simulink model "Mdl_wFuelLidOpen"  (R2024b)
settings: Solver=FixedStepDiscrete  StartTime=0.0  StopTime=10.0  FixedStep=0.1  RelTol=1e-3  EnableMultiTasking=on
values from neighbouring files (symbols this model uses):
  FUEL_CAN_SIG_VAL_ONE = mpt.Parameter    [Mdl_wFuelLidOpen_dd.m]
  FUEL_PAYLOAD_INVALID_VALUE = mpt.Parameter    [Mdl_wFuelLidOpen_dd.m]
undefined symbols (not defined in the file or in its folder): CLUSTER_INACTIVE, eSIGNAL_MISSING, eSIGNAL_NEVER_RECEIVED, eWarningIn, IgnOff, pJustRcvdStatus, RxCan_SignalClearJustRcvdStatus, RxCan_SignalGetJustRcvdStatus, RxCan_SignalInvalidProcessingControl, RxCan_SignalMissingProcessingControl, RxCan_SignalNRProcessingControl, SignalId, Status, tRxSignalId_type_instance, tRxSignalJustRcvdStatus_type_instance, tRxSignalStatus_type_instance, UI_WARNING_EVENT_NONE, UI_WARNING_STATUS_OFF, UI_WARNING_STATUS_ON, UpdateWarningStatus, WarningCurEvent, WarningCurId, WarningCurStatus, WarningEvent_type_instance, WarningId_type_instance, WarningPayload, WarningStatus_type_instance, WRN_NORM_FUECAP_02
libraries: simulink x1
settings Model: Creator=AELANGO6  LastModifiedBy=AELANGO6
settings DataIOCC: SaveOutput=off
settings OptimizationCC: DefaultParameterBehavior=Inlined  EnhancedBackFolding=on  PassReuseOutputArgsAs=Individual arguments  ZeroExternalMemoryAtStartup=off  ZeroInternalMemoryAtStartup=off  MaxStackSize=750  RemoveLocalVariableInitialization=off  OptimizeBlockOrder=speed  DifferentSizesBufferReuse=on  OptimizationCustomize=off  EfficientTunableParamExpr=on
settings DebuggingCC: ParameterTunabilityLossMsg=error
settings SFSimCC: MATLABDynamicMemAlloc=off
settings RTWCC: Description=AUTOSAR  SystemTargetFile=autosar.tlc  GenCodeOnly=on  TemplateMakefile=ert_default_tmf  PortableWordSizes=on  DataTypeReplacement=CDataTypesFixedWidth
settings CodeAppCC: ForceParamTrailComments=on  IgnoreCustomStorageClasses=off  OperatorAnnotations=on  SimulinkDataObjDesc=on  SFDataObjDesc=on  InsertBlockDesc=on
settings STFCustomTargetCC: TargetLangStandard=C99 (ISO)  MultiwordLength=256  ParMdlRefBuildCompliant=on  CompOptLevelCompliant=on  IncludeMdlTerminateFcn=off  CombineOutputUpdateFcns=on  SuppressErrorStatus=on  ERTCustomFileBanners=on  SupportNonFinite=off  SupportComplex=off  SupportContinuousTime=off  SupportNonInlinedSFcns=off  RemoveResetFunc=on  ParenthesesLevel=Maximum  CastingMode=Standards  MATLABClassNameForMDSCustomization=Simulink.SoftwareTarget.ERTCustomization  AutosarCompliant=on  UseToolchainInfoCompliant=on  LookupTableObjectStructAxisOrder=2,1,3,4,...  LUTObjectStructOrderEvenSpacing=Size,Table,Breakpoints  SystemTargetFile=autosar.tlc
settings ERTTargetCC: TargetLangStandard=C99 (ISO)  ConcurrentExecutionCompliant=off  IncludeMdlTerminateFcn=off  SuppressErrorStatus=on  SupportNonFinite=off  SupportComplex=off  ParenthesesLevel=Maximum  CastingMode=Standards  ModelStepFunctionPrototypeControlCompliant=off  CPPClassGenCompliant=off  AutosarCompliant=on  LookupTableObjectStructAxisOrder=2,1,3,4,...  LUTObjectStructOrderEvenSpacing=Size,Table,Breakpoints  ERTCustomFileTemplate=example_file_process.tlc  ERTFilePackagingFormat=CompactWithDataFile  BooleanTrueId=TRUE  BooleanFalseId=FALSE

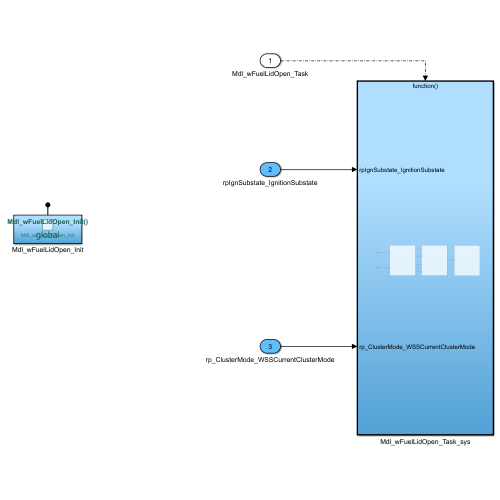
[thumbnail: Simulink's stored preview of the top-level diagram]
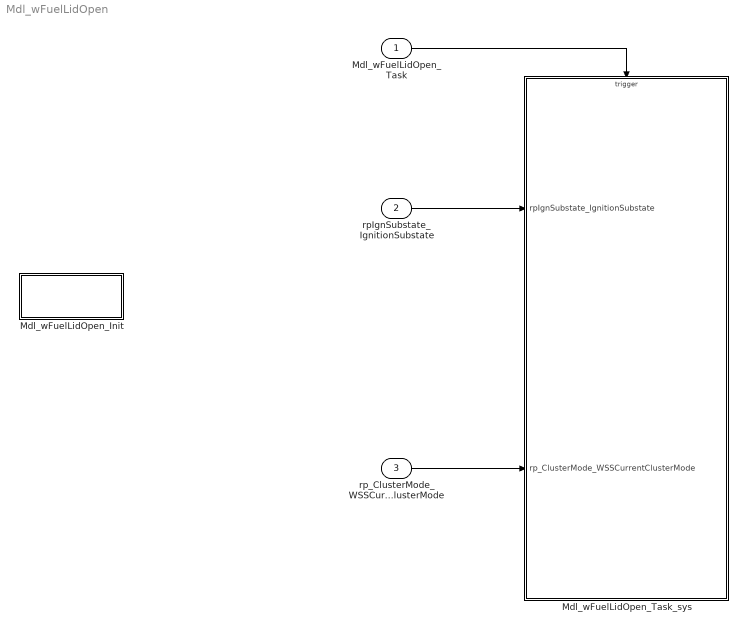
== system Mdl_wFuelLidOpen ==
  Mdl_wFuelLidOpen_Task : Inport  SampleTime=0.1  OutputFunctionCall=on
  rpIgnSubstate_IgnitionSubstate : Inport  Port=2  OutDataTypeStr=IgntionSubstateType  PortDimensions=1
  rp_ClusterMode_WSSCurrentClusterMode : Inport  Port=3  OutDataTypeStr=ClusterModes  PortDimensions=1
  Mdl_wFuelLidOpen_Init : Subsystem  TreatAsAtomicUnit=on
  Mdl_wFuelLidOpen_Task_sys : Subsystem  TreatAsAtomicUnit=on
  wires:
  Mdl_wFuelLidOpen_Task/1 -> Mdl_wFuelLidOpen_Task_sys/Trigger
  rpIgnSubstate_IgnitionSubstate/1 -> Mdl_wFuelLidOpen_Task_sys/1(rpIgnSubstate_IgnitionSubstate)
  rp_ClusterMode_WSSCurrentClusterMode/1 -> Mdl_wFuelLidOpen_Task_sys/2(rp_ClusterMode_WSSCurrentClusterMode)

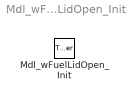
== system Mdl_wFuelLidOpen/Mdl_wFuelLidOpen_Init ==
  Mdl_wFuelLidOpen_Init : TriggerPort  TriggerType=function-call  IsSimulinkFunction=on  FunctionName=Mdl_wFuelLidOpen_Init  VariantControl=(inherit)

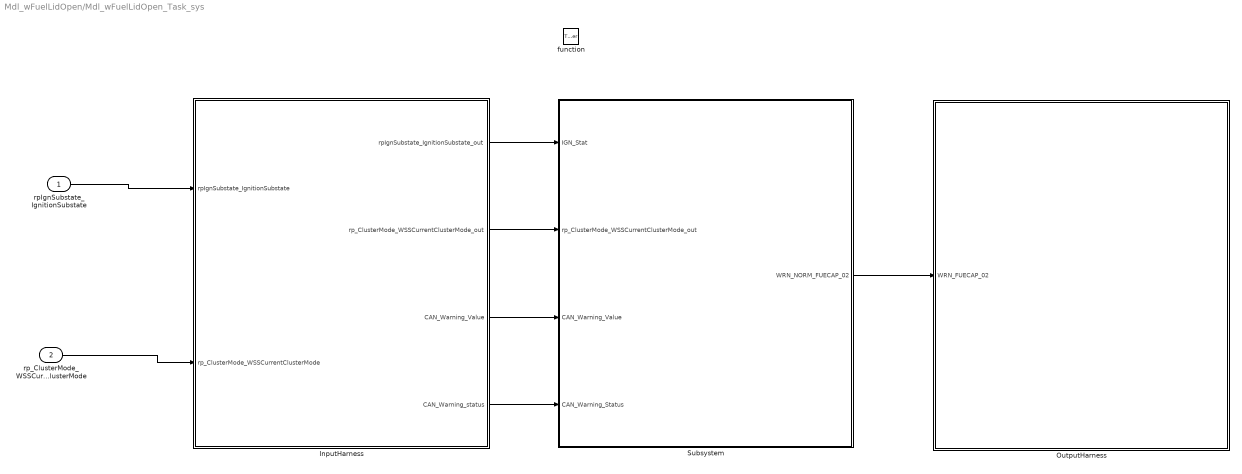
== system Mdl_wFuelLidOpen/Mdl_wFuelLidOpen_Task_sys ==
  rpIgnSubstate_IgnitionSubstate : Inport  OutDataTypeStr=IgntionSubstateType  PortDimensions=1
  rp_ClusterMode_WSSCurrentClusterMode : Inport  Port=2  OutDataTypeStr=ClusterModes  PortDimensions=1
  function : TriggerPort  TriggerType=function-call  VariantControl=(inherit)  SampleTimeType=periodic  SampleTime=-1
  InputHarness : Subsystem  Variant=on
  OutputHarness : Subsystem  Variant=on
  Subsystem : Subsystem
  wires:
  rpIgnSubstate_IgnitionSubstate/1 -> InputHarness/1(rpIgnSubstate_IgnitionSubstate)
  rp_ClusterMode_WSSCurrentClusterMode/1 -> InputHarness/2(rp_ClusterMode_WSSCurrentClusterMode)
  InputHarness/3(CAN_Warning_Value) -> Subsystem/3(CAN_Warning_Value)
  InputHarness/4(CAN_Warning_status) -> Subsystem/4(CAN_Warning_Status)
  InputHarness/2(rp_ClusterMode_WSSCurrentClusterMode_out) -> Subsystem/2(rp_ClusterMode_WSSCurrentClusterMode_out)
  InputHarness/1(rpIgnSubstate_IgnitionSubstate_out) -> Subsystem/1(IGN_Stat)
  Subsystem/1(WRN_NORM_FUECAP_02) -> OutputHarness/1(WRN_FUECAP_02)

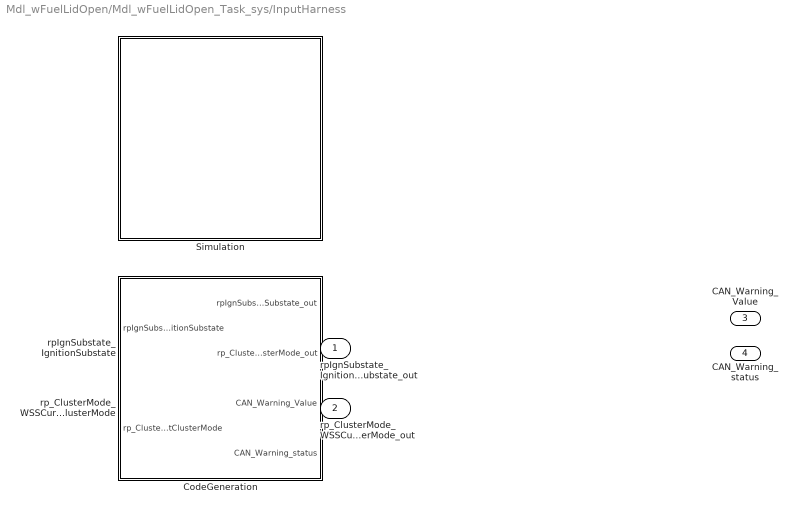
== system Mdl_wFuelLidOpen/Mdl_wFuelLidOpen_Task_sys/InputHarness ==
  rpIgnSubstate_IgnitionSubstate : Inport  OutDataTypeStr=IgntionSubstateType  PortDimensions=1
  rp_ClusterMode_WSSCurrentClusterMode : Inport  Port=2  OutDataTypeStr=ClusterModes  PortDimensions=1
  CodeGeneration : Subsystem  VariantControl=CODEGENERATION
  Simulation : Subsystem  VariantControl=SIMULATION
  rpIgnSubstate_IgnitionSubstate_out : Outport  OutDataTypeStr=IgntionSubstateType  PortDimensions=1
  rp_ClusterMode_WSSCurrentClusterMode_out : Outport  Port=2  OutDataTypeStr=ClusterModes  PortDimensions=1
  CAN_Warning_Value : Outport  Port=3  OutDataTypeStr=uint8  VectorParamsAs1DForOutWhenUnconnected=off
  CAN_Warning_status : Outport  Port=4  OutDataTypeStr=uint8  VectorParamsAs1DForOutWhenUnconnected=off

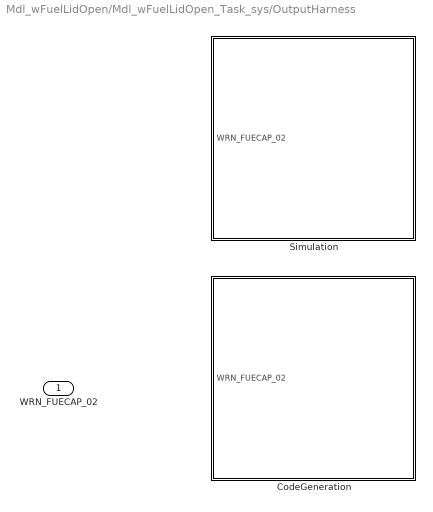
== system Mdl_wFuelLidOpen/Mdl_wFuelLidOpen_Task_sys/OutputHarness ==
  WRN_FUECAP_02 : Inport
  CodeGeneration : Subsystem  VariantControl=CODEGENERATION
  Simulation : Subsystem  VariantControl=SIMULATION

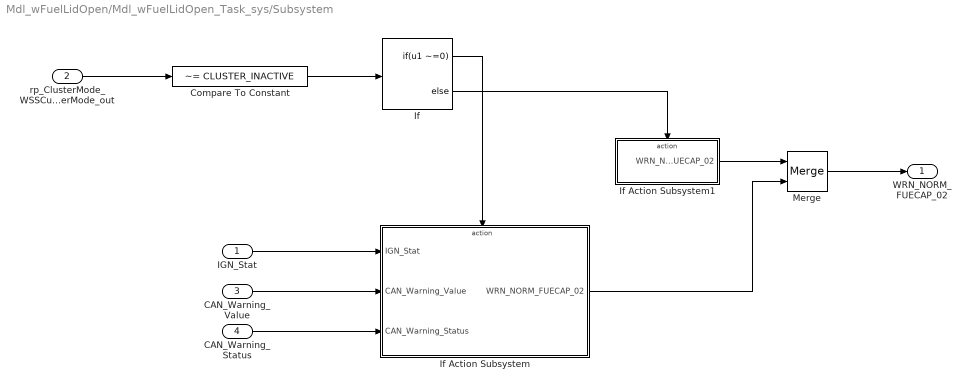
== system Mdl_wFuelLidOpen/Mdl_wFuelLidOpen_Task_sys/Subsystem ==
  IGN_Stat : Inport
  rp_ClusterMode_WSSCurrentClusterMode_out : Inport  Port=2
  CAN_Warning_Value : Inport  Port=3
  CAN_Warning_Status : Inport  Port=4
  Compare To Constant : simulink/Logic and Bit Operations/Compare To Constant  relop=~=  const=CLUSTER_INACTIVE  OutDataTypeStr=boolean
  If : If  IfExpression=u1 ~=0
  If Action Subsystem : Subsystem  TreatAsAtomicUnit=on
  If Action Subsystem1 : Subsystem  TreatAsAtomicUnit=on
  Merge : Merge
  WRN_NORM_FUECAP_02 : Outport  VectorParamsAs1DForOutWhenUnconnected=off
  wires:
  Compare To Constant/1 -> If/1
  rp_ClusterMode_WSSCurrentClusterMode_out/1 -> Compare To Constant/1
  IGN_Stat/1 -> If Action Subsystem/1(IGN_Stat)
  CAN_Warning_Value/1 -> If Action Subsystem/2(CAN_Warning_Value)
  CAN_Warning_Status/1 -> If Action Subsystem/3(CAN_Warning_Status)
  If/1 -> If Action Subsystem/Action
  If/2 -> If Action Subsystem1/Action
  Merge/1 -> WRN_NORM_FUECAP_02/1
  If Action Subsystem/1(WRN_NORM_FUECAP_02) -> Merge/2
  If Action Subsystem1/1(WRN_NORM_FUECAP_02) -> Merge/1

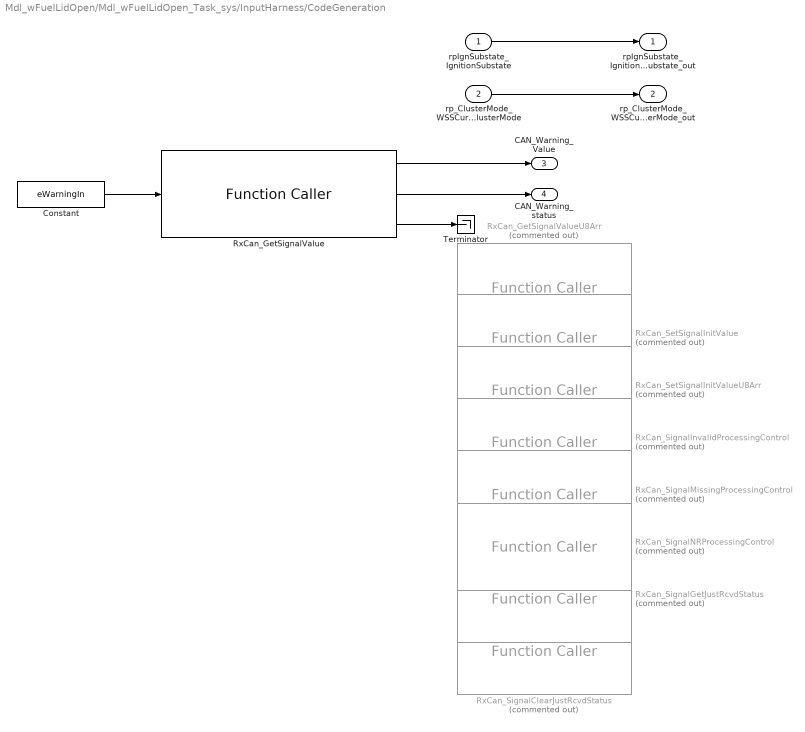
== system Mdl_wFuelLidOpen/Mdl_wFuelLidOpen_Task_sys/InputHarness/CodeGeneration ==
  rpIgnSubstate_IgnitionSubstate : Inport  OutDataTypeStr=IgntionSubstateType  PortDimensions=1
  rp_ClusterMode_WSSCurrentClusterMode : Inport  Port=2  OutDataTypeStr=ClusterModes  PortDimensions=1
  Constant : Constant  Value=eWarningIn
  RxCan_GetSignalValue : FunctionCaller  FunctionPrototype=[pSignalValue,pSignalStatus,error_status] = RxCan_GetSignalValue(SignalId)  InputArgumentSpecifications=tRxSignalId_type_instance(1)  OutputArgumentSpecifications=uint8(1) ,tRxSignalStatus_type_instance(1) ,uint8(1)
  RxCan_GetSignalValueU8Arr : FunctionCaller  Commented=on  FunctionPrototype=[pSignalValue,pSignalStatus,pSignalLength,error_status] = RxCan_GetSignalValueU8Arr(SignalId)  InputArgumentSpecifications=tRxSignalId_type_instance(1)  OutputArgumentSpecifications=uint8(1) ,tRxSignalStatus_type_instance(1) ,uint32(1) ,uint8(1)
  RxCan_SetSignalInitValue : FunctionCaller  Commented=on  FunctionPrototype=[pSignalValue,error_status] = RxCan_SetSignalInitValue(SignalId)  InputArgumentSpecifications=tRxSignalId_type_instance(1)  OutputArgumentSpecifications=uint8(1) ,uint8(1)
  RxCan_SetSignalInitValueU8Arr : FunctionCaller  Commented=on  FunctionPrototype=[pSignaValue,pSignalLength,error_status] = RxCan_SetSignalInitValueU8Arr(SignalId)  InputArgumentSpecifications=tRxSignalId_type_instance(1)  OutputArgumentSpecifications=uint8(1) ,uint32(1) ,uint8(1)
  RxCan_SignalClearJustRcvdStatus : FunctionCaller  Commented=on  FunctionPrototype=RxCan_SignalClearJustRcvdStatus(SignalId)  InputArgumentSpecifications=tRxSignalId_type_instance(1)  OutputArgumentSpecifications=<Enter example>
  RxCan_SignalGetJustRcvdStatus : FunctionCaller  Commented=on  FunctionPrototype=RxCan_SignalGetJustRcvdStatus(SignalId,pJustRcvdStatus)  InputArgumentSpecifications=tRxSignalId_type_instance(1) ,tRxSignalJustRcvdStatus_type_instance(1)  OutputArgumentSpecifications=<Enter example>
  RxCan_SignalInvalidProcessingControl : FunctionCaller  Commented=on  FunctionPrototype=RxCan_SignalInvalidProcessingControl(SignalId,Status)  InputArgumentSpecifications=tRxSignalId_type_instance(1) ,boolean(1)  OutputArgumentSpecifications=<Enter example>
  RxCan_SignalMissingProcessingControl : FunctionCaller  Commented=on  FunctionPrototype=RxCan_SignalMissingProcessingControl(SignalId,Status)  InputArgumentSpecifications=tRxSignalId_type_instance(1) ,boolean(1)  OutputArgumentSpecifications=<Enter example>
  RxCan_SignalNRProcessingControl : FunctionCaller  Commented=on  FunctionPrototype=RxCan_SignalNRProcessingControl(SignalId,Status)  InputArgumentSpecifications=tRxSignalId_type_instance(1) ,boolean(1)  OutputArgumentSpecifications=<Enter example>
  Terminator : Terminator
  rpIgnSubstate_IgnitionSubstate_out : Outport  OutDataTypeStr=IgntionSubstateType  PortDimensions=1
  rp_ClusterMode_WSSCurrentClusterMode_out : Outport  Port=2  OutDataTypeStr=ClusterModes  PortDimensions=1
  CAN_Warning_Value : Outport  Port=3  OutDataTypeStr=uint8  VectorParamsAs1DForOutWhenUnconnected=off
  CAN_Warning_status : Outport  Port=4  OutDataTypeStr=uint8  VectorParamsAs1DForOutWhenUnconnected=off
  wires:
  rpIgnSubstate_IgnitionSubstate/1 -> rpIgnSubstate_IgnitionSubstate_out/1
  rp_ClusterMode_WSSCurrentClusterMode/1 -> rp_ClusterMode_WSSCurrentClusterMode_out/1
  RxCan_GetSignalValue/2 -> CAN_Warning_status/1
  RxCan_GetSignalValue/1 -> CAN_Warning_Value/1
  RxCan_GetSignalValue/3 -> Terminator/1
  Constant/1 -> RxCan_GetSignalValue/1

== system Mdl_wFuelLidOpen/Mdl_wFuelLidOpen_Task_sys/InputHarness/Simulation ==

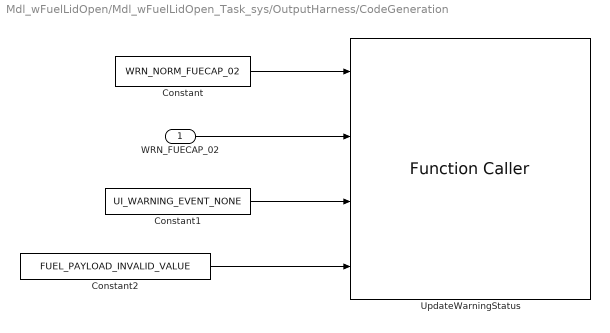
== system Mdl_wFuelLidOpen/Mdl_wFuelLidOpen_Task_sys/OutputHarness/CodeGeneration ==
  WRN_FUECAP_02 : Inport  OutDataTypeStr=uint8
  Constant : Constant  Value=WRN_NORM_FUECAP_02  OutDataTypeStr=Inherit: Inherit via back propagation
  Constant1 : Constant  Value=UI_WARNING_EVENT_NONE
  Constant2 : Constant  Value=FUEL_PAYLOAD_INVALID_VALUE  OutDataTypeStr=uint32
  UpdateWarningStatus : FunctionCaller  FunctionPrototype=UpdateWarningStatus(WarningCurId,WarningCurStatus,WarningCurEvent,WarningPayload)  InputArgumentSpecifications=WarningId_type_instance(1) ,WarningStatus_type_instance(1) ,WarningEvent_type_instance(1) ,uint32(1)  OutputArgumentSpecifications=<Enter example>
  wires:
  Constant2/1 -> UpdateWarningStatus/4
  Constant/1 -> UpdateWarningStatus/1
  Constant1/1 -> UpdateWarningStatus/3
  WRN_FUECAP_02/1 -> UpdateWarningStatus/2

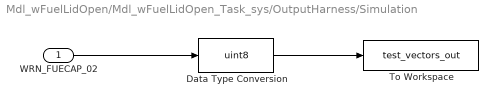
== system Mdl_wFuelLidOpen/Mdl_wFuelLidOpen_Task_sys/OutputHarness/Simulation ==
  WRN_FUECAP_02 : Inport
  Data Type Conversion : DataTypeConversion  OutDataTypeStr=uint8  SaturateOnIntegerOverflow=off  RndMeth=Floor
  To Workspace : ToWorkspace  VariableName=test_vectors_out  SampleTime=-1
      settings: Save2DSignal=2-D array (concatenate along first dimension)
  wires:
  Data Type Conversion/1 -> To Workspace/1
  WRN_FUECAP_02/1 -> Data Type Conversion/1

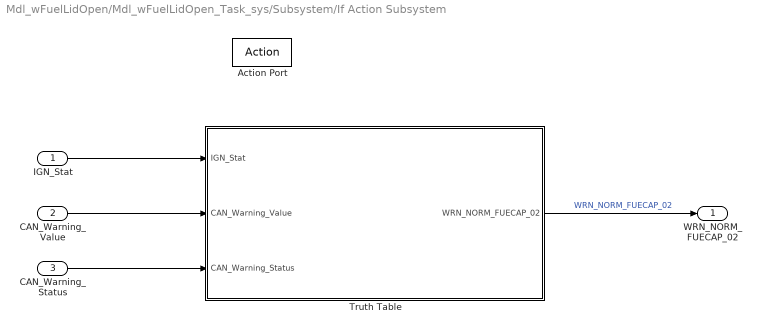
== system Mdl_wFuelLidOpen/Mdl_wFuelLidOpen_Task_sys/Subsystem/If Action Subsystem ==
  IGN_Stat : Inport
  CAN_Warning_Value : Inport  Port=2
  CAN_Warning_Status : Inport  Port=3
  Action Port : ActionPort  ActionPortLabel=if(u1 ~=0)
  Truth Table : Truth Table  TreatAsAtomicUnit=on
  WRN_NORM_FUECAP_02 : Outport  VectorParamsAs1DForOutWhenUnconnected=off
  wires:
  CAN_Warning_Status/1 -> Truth Table/3(CAN_Warning_Status)
  IGN_Stat/1 -> Truth Table/1(IGN_Stat)
  CAN_Warning_Value/1 -> Truth Table/2(CAN_Warning_Value)
  Truth Table/1(WRN_NORM_FUECAP_02) -> WRN_NORM_FUECAP_02/1  "WRN_NORM_FUECAP_02"

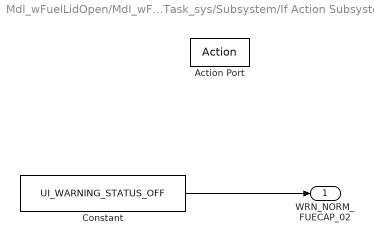
== system Mdl_wFuelLidOpen/Mdl_wFuelLidOpen_Task_sys/Subsystem/If Action Subsystem1 ==
  Action Port : ActionPort  ActionPortLabel=else
  Constant : Constant  Value=UI_WARNING_STATUS_OFF  SampleTime=-1
  WRN_NORM_FUECAP_02 : Outport  VectorParamsAs1DForOutWhenUnconnected=off
  wires:
  Constant/1 -> WRN_NORM_FUECAP_02/1

== matlab function Mdl_wFuelLidOpen/Mdl_wFuelLidOpen_Task_sys/Subsystem/If Action Subsystem/Truth Table ==
  data: IGN_Stat input; WRN_NORM_FUECAP_02 output; CAN_Warning_Value input; CAN_Warning_Status input; IgnOff parameter; eSIGNAL_MISSING parameter; eSIGNAL_NEVER_RECEIVED parameter; UI_WARNING_STATUS_ON parameter; UI_WARNING_STATUS_OFF parameter; FUEL_CAN_SIG_VAL_ONE parameter
function WRN_NORM_FUECAP_02 = fcn(IGN_Stat, CAN_Warning_Value, CAN_Warning_Status, IgnOff, eSIGNAL_MISSING, eSIGNAL_NEVER_RECEIVED, UI_WARNING_STATUS_ON, UI_WARNING_STATUS_OFF, FUEL_CAN_SIG_VAL_ONE)

aVarTruthTableCondition_1 = false;
aVarTruthTableCondition_2 = false;


% IGN OF condition

aVarTruthTableCondition_1 = logical((IGN_Stat == IgnOff) || (CAN_Warning_Status== eSIGNAL_MISSING) ||  (CAN_Warning_Status== eSIGNAL_NEVER_RECEIVED));

% CAN Data Received

aVarTruthTableCondition_2 = logical(CAN_Warning_Value==FUEL_CAN_SIG_VAL_ONE);

if (aVarTruthTableCondition_1)
    aFcnTruthTableAction_1();
elseif (aVarTruthTableCondition_2)
    aFcnTruthTableAction_2();
else % Default
    aFcnTruthTableAction_1();
end

function aFcnTruthTableAction_1()

% WRN_NORM_FUELCAP is OFF

WRN_NORM_FUECAP_02 =UI_WARNING_STATUS_OFF;

function aFcnTruthTableAction_2()

% WRN_NORM_FUELCAP  is ON

WRN_NORM_FUECAP_02= UI_WARNING_STATUS_ON;
